simulink model "EvReferenceApplication"  (R2024b)
settings: Solver=ode23tb  StartTime=0  StopTime=2474  RelTol=1e-3  EnableMultiTasking=on
undefined symbols (not defined in the file or in its folder): SRE
undefined symbols (not defined in the file): FTP75
libraries: autolibshared x2, simulink x1, autolibutils x1
settings Model: DataDictionary=BMS_Software_DD.sldd  ModifiedByFormat=The MathWorks, Inc.  PauseTimes=0  Creator=The MathWorks, Inc.  LastModifiedBy=The MathWorks, Inc.
settings SolverCC: ZeroCrossAlgorithm=Adaptive  AlgebraicLoopSolver=TrustRegion  AutoInsertRateTranBlk=on  DecoupledContinuousIntegration=on  MinimalZcImpactIntegration=on  MaxZcPerStep=1
settings DataIOCC: SaveOutput=off  DSMLogging=off  SaveTime=off  ReturnWorkspaceOutputs=off  ReturnWorkspaceOutputsName=tp18ed42d9_4bab_49d7_8847_516cfb0e46d8
settings DebuggingCC: UnderspecifiedInitializationDetection=Classic  MergeDetectMultiDrivingBlocksExec=none  IgnoredZcDiagnostic=none  ParameterPrecisionLossMsg=none  UnconnectedInputMsg=warning  UnconnectedOutputMsg=warning  UnconnectedLineMsg=warning  PregeneratedLibrarySubsystemCodeDiagnostic=none  SubsystemReferenceDiagnosticForUnitTest=warning  ArithmeticOperatorsInVariantConditions=warning
settings ModelReferenceCC: UpdateModelReferenceTargets=IfOutOfDate  EnableRefExpFcnMdlSchedulingChecks=on  ModelReferenceMinAlgLoopOccurrences=on  PropagateSignalLabelsOutOfModel=off
settings SFSimCC: SimUseLocalCustomCode=off
settings RTWCC: RTWUseLocalCustomCode=off  GPUComputeCapability=3.5  DLArmComputeVersion=19.05
settings CodeAppCC: StateflowObjectComments=on
settings GRTTargetCC: TargetLangStandard=C89/C90 (ANSI)
settings ConfigComp: CovMetricSettings=dsw  CovSaveCumulativeToWorkspaceVar=on  CovSaveSingleToWorkspaceVar=on  CovExternalEMLEnable=off
settings SimscapeCC: SimscapeLogSimulationStatistics=on  SimscapeLogToSDI=on  SimscapeLogOpenViewer=on  SimscapeLogLimitData=off

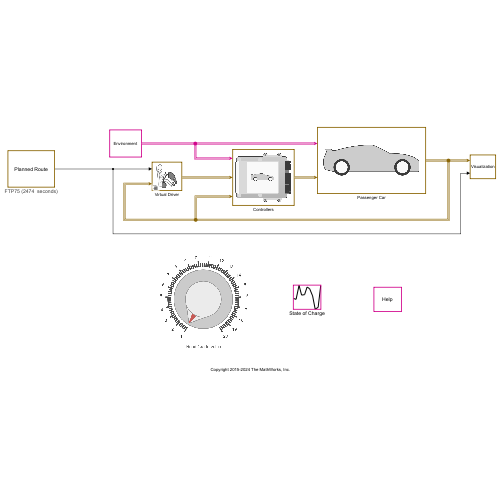
[thumbnail: Simulink's stored preview of the top-level diagram]
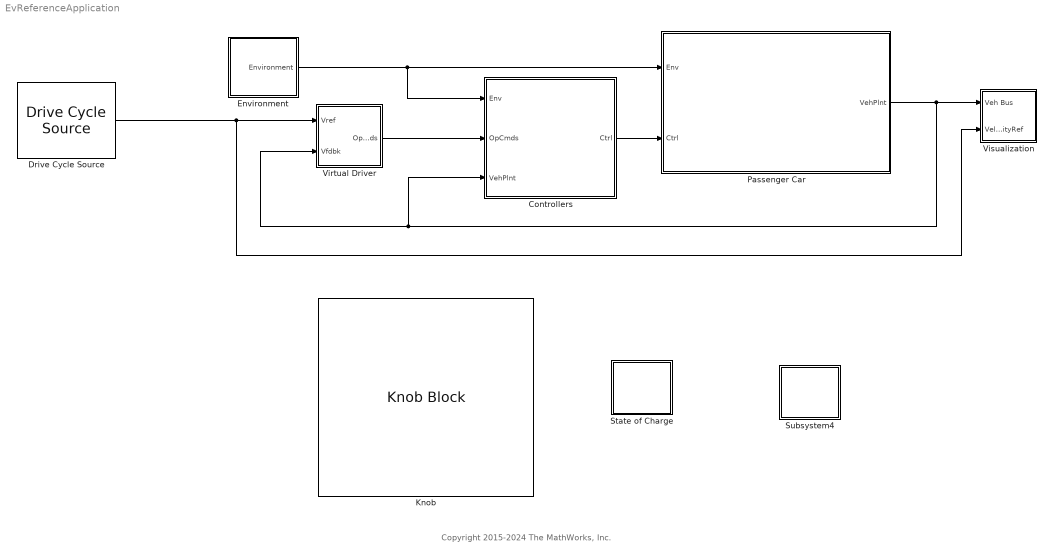
== system EvReferenceApplication ==
  note: Copyright 2015-2024 The MathWorks, Inc.
  Controllers : Subsystem
      mask Display: image('SystemControllers.png','center')
  Drive Cycle Source : autolibshared/Drive Cycle Source  cycleVar=FTP75  fileVar=L:\Bauto\matlab\test\toolbox\shared\autoblks\scenario\adac.txt  tfinal="2474  seconds"  cycleRepeat=off  outAccPort=off  outGearPort=off  gearList=No gear data  t_wot1=1  xdot_woto=0  xdot_wot1=26.8*1.1  t_wot2=30  xdot_wot2=0  t_wotend=40  srcUnit=m/s  outUnit=m/s  srcAccUnit=m/s/s  outAccUnit=m/s^2  dt=0  aMode=1  faultOption=off  velBnd=2  velBndUnit=mph  inUnit=m/s  timeBnd=1  failOption=off  stopSim=off  maxFaultCnt=10  maxFaultTime=2  maxTotFaultTime=15  traceOption=off  dtTrace=1  traceWindow=10  lastDCname=UDDS  lastOutUnit=mph  lastDT=0  lastTB=1  lastSB=2  forceCalcBound=off  mask(Drive Cycle Source){cycleVar=FTP75}
      mask prompts: cycleVar "autoblks_shared:autoblkDriveCycleSource:blkPrm_cycleVar"
      mask TypeOptions cycleVar: cycleVar
      mask DialogControl cycleVar Prompt: Drive cycle source:
      mask Display: fprintf('Planned Route');
  Environment : Subsystem
      mask Display: disp(getString(message('autoblks:autoblkVehMask:environ')))
  Knob : KnobBlock  LabelPosition=Bottom  ScaleMin=1  ScaleMax=20
  Passenger Car : Subsystem
      mask Display: image('PassengerVehicle.png','center')
  State of Charge : Subsystem
      settings: OpenFcn=open_system('EvReferenceApplication/Visualization/Scope');
      mask Display: plot(0:5:50, [.5000    0.4799    0.9047    0.6099    0.6177    0.8594    0.8055    0.5767    0.1829    0.2399    0.8865]);
  Subsystem4 : Subsystem
      settings: OpenFcn=helpview([docroot,'/toolbox/autoblks/helptargets.map'], 'ev_refapp')
      mask Display: disp(getString(message('autoblks:autoblkVehMask:help')))
  Virtual Driver : Subsystem  Variant=on  VariantControlMode=label  VariantControl=Variant1  LabelModeActiveChoice=0
      mask Display:
      | if strcmp('1',get_param(gcb,'ActiveVariant'))
      |     disp('Open Loop')
      | else
      |     image('LongitudinalDriver.png','center');
      | end
  Visualization : Subsystem
      mask Display: disp(getString(message('autoblks:autoblkVehMask:visual')))
  wires:
  Virtual Driver/1(" OpCmds") -> Controllers/2(OpCmds)
  Drive Cycle Source/1 -> Virtual Driver/1("Vref "), Visualization/2(VelocityRef)
  Environment/1(Environment) -> Controllers/1(Env), Passenger Car/1(Env)
  Controllers/1(Ctrl) -> Passenger Car/2(Ctrl)
  Passenger Car/1(VehPlnt) -> Visualization/1(Veh Bus), Virtual Driver/2("Vfdbk "), Controllers/3(VehPlnt)

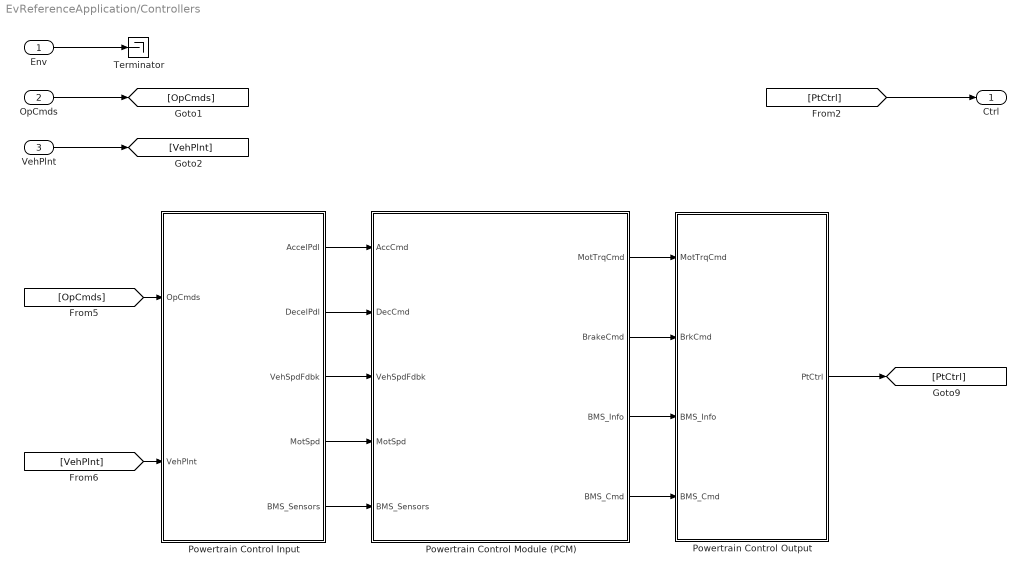
== system EvReferenceApplication/Controllers ==
  Env : Inport
  OpCmds : Inport  Port=2
  VehPlnt : Inport  Port=3
  Powertrain Control Input : Subsystem
  Powertrain Control Module (PCM) : Subsystem
  Powertrain Control Output : Subsystem
  Terminator : Terminator
  Ctrl : Outport  VectorParamsAs1DForOutWhenUnconnected=off
  wires:
  [PtCtrl] -> Ctrl/1
  Env/1 -> Terminator/1
  [OpCmds] -> Powertrain Control Input/1(OpCmds)
  Powertrain Control Output/1(PtCtrl) -> [PtCtrl]
  [VehPlnt] -> Powertrain Control Input/2(VehPlnt)
  VehPlnt/1 -> [VehPlnt]
  OpCmds/1 -> [OpCmds]
  Powertrain Control Input/1(AccelPdl) -> Powertrain Control Module (PCM)/1(AccCmd)
  Powertrain Control Input/2(DecelPdl) -> Powertrain Control Module (PCM)/2(DecCmd)
  Powertrain Control Input/3(VehSpdFdbk) -> Powertrain Control Module (PCM)/3(VehSpdFdbk)
  Powertrain Control Input/4(MotSpd) -> Powertrain Control Module (PCM)/4(MotSpd)
  Powertrain Control Module (PCM)/1(MotTrqCmd) -> Powertrain Control Output/1(MotTrqCmd)
  Powertrain Control Module (PCM)/2(BrakeCmd) -> Powertrain Control Output/2(BrkCmd)
  Powertrain Control Input/5(BMS_Sensors) -> Powertrain Control Module (PCM)/5(BMS_Sensors)
  Powertrain Control Module (PCM)/3(BMS_Info) -> Powertrain Control Output/3(BMS_Info)
  Powertrain Control Module (PCM)/4(BMS_Cmd) -> Powertrain Control Output/4(BMS_Cmd)

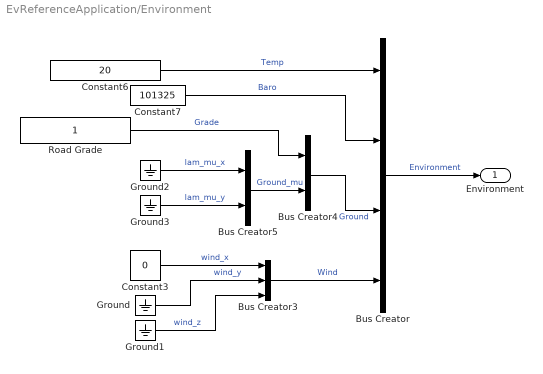
== system EvReferenceApplication/Environment ==
  Bus Creator : BusCreator  Inputs=4
  Bus Creator3 : BusCreator  Inputs=3
  Bus Creator4 : BusCreator  Inputs=2
  Bus Creator5 : BusCreator  Inputs=2
  Constant3 : Constant  Value=0
  Constant6 : Constant  Value=20
  Constant7 : Constant  Value=101325
  Ground{,1..3} (4 alike) : Ground
  Road Grade : Constant
      settings: AttributesFormatString=%<Name>
  Environment : Outport  VectorParamsAs1DForOutWhenUnconnected=off
  wires:
  Ground2/1 -> Bus Creator5/1  "lam_mu_x"
  Ground3/1 -> Bus Creator5/2  "lam_mu_y"
  Bus Creator5/1 -> Bus Creator4/2  "Ground_mu"
  Bus Creator4/1 -> Bus Creator/3  "Ground"
  Bus Creator3/1 -> Bus Creator/4  "Wind"
  Constant3/1 -> Bus Creator3/1  "wind_x"
  Ground/1 -> Bus Creator3/2  "wind_y"
  Ground1/1 -> Bus Creator3/3  "wind_z"
  Constant6/1 -> Bus Creator/1  "Temp"
  Road Grade/1 -> Bus Creator4/1  "Grade"
  Bus Creator/1 -> Environment/1  "Environment"
  Constant7/1 -> Bus Creator/2  "Baro"

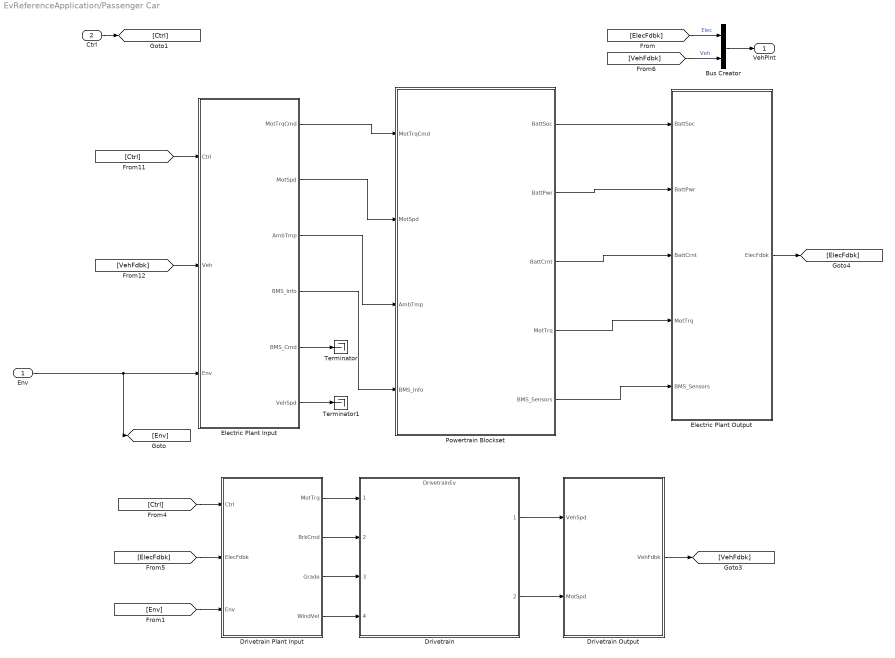
== system EvReferenceApplication/Passenger Car ==
  Env : Inport
  Ctrl : Inport  Port=2
  Bus Creator : BusCreator  Inputs=2
  Drivetrain : ModelReference  ModelNameDialog=DrivetrainEv.slx  ModelReferenceVersion=10.0
  Drivetrain Output : Subsystem
  Drivetrain Plant Input : Subsystem
  Electric Plant Input : Subsystem
  Electric Plant Output : Subsystem
  Powertrain Blockset : Subsystem  VariantControl=Powertrain Blockset
  Terminator : Terminator
  Terminator1 : Terminator
  VehPlnt : Outport  VectorParamsAs1DForOutWhenUnconnected=off
  wires:
  Ctrl/1 -> [Ctrl]
  Env/1 -> [Env], Electric Plant Input/3(Env)
  [Ctrl] -> Drivetrain Plant Input/1(Ctrl)
  Bus Creator/1 -> VehPlnt/1
  [VehFdbk] -> Bus Creator/2  "Veh"
  Drivetrain Output/1(VehFdbk) -> [VehFdbk]
  Electric Plant Output/1(ElecFdbk) -> [ElecFdbk]
  [ElecFdbk] -> Bus Creator/1  "Elec"
  [Ctrl] -> Electric Plant Input/1(Ctrl)
  [ElecFdbk] -> Drivetrain Plant Input/2(ElecFdbk)
  [VehFdbk] -> Electric Plant Input/2(Veh)
  Drivetrain Plant Input/2(BrkCmd) -> Drivetrain/2
  Drivetrain Plant Input/1(MotTrq) -> Drivetrain/1
  Drivetrain/2 -> Drivetrain Output/2(MotSpd)
  Drivetrain/1 -> Drivetrain Output/1(VehSpd)
  [Env] -> Drivetrain Plant Input/3(Env)
  Drivetrain Plant Input/3(Grade) -> Drivetrain/3
  Drivetrain Plant Input/4(WindVel) -> Drivetrain/4
  Electric Plant Input/1(MotTrqCmd) -> Powertrain Blockset/1(MotTrqCmd)
  Powertrain Blockset/2(BattPwr) -> Electric Plant Output/2(BattPwr)
  Electric Plant Input/2(MotSpd) -> Powertrain Blockset/2(MotSpd)
  Electric Plant Input/3(AmbTmp) -> Powertrain Blockset/3(AmbTmp)
  Electric Plant Input/4(BMS_Info) -> Powertrain Blockset/4(BMS_Info)
  Powertrain Blockset/1(BattSoc) -> Electric Plant Output/1(BattSoc)
  Powertrain Blockset/3(BattCrnt) -> Electric Plant Output/3(BattCrnt)
  Powertrain Blockset/4(MotTrq) -> Electric Plant Output/4(MotTrq)
  Powertrain Blockset/5(BMS_Sensors) -> Electric Plant Output/5(BMS_Sensors)
  Electric Plant Input/5(BMS_Cmd) -> Terminator/1
  Electric Plant Input/6(VehSpd) -> Terminator1/1

== system EvReferenceApplication/State of Charge ==

== system EvReferenceApplication/Subsystem4 ==

== system EvReferenceApplication/Virtual Driver ==
  note: To switch variants, right-click on this subsystem (from one level above) and chose:
      | Variant, Active choice, <your selection>
  "Vref " : Inport
  "Vfdbk " : Inport  Port=2
  Longitudinal Driver : Subsystem  VariantControl=0
      mask Display: image('LongitudinalDriver.png', 'center')
  Open Loop : Subsystem  VariantControl=1
      mask Display: disp('Open Loop')
  " OpCmds" : Outport  VectorParamsAs1DForOutWhenUnconnected=off

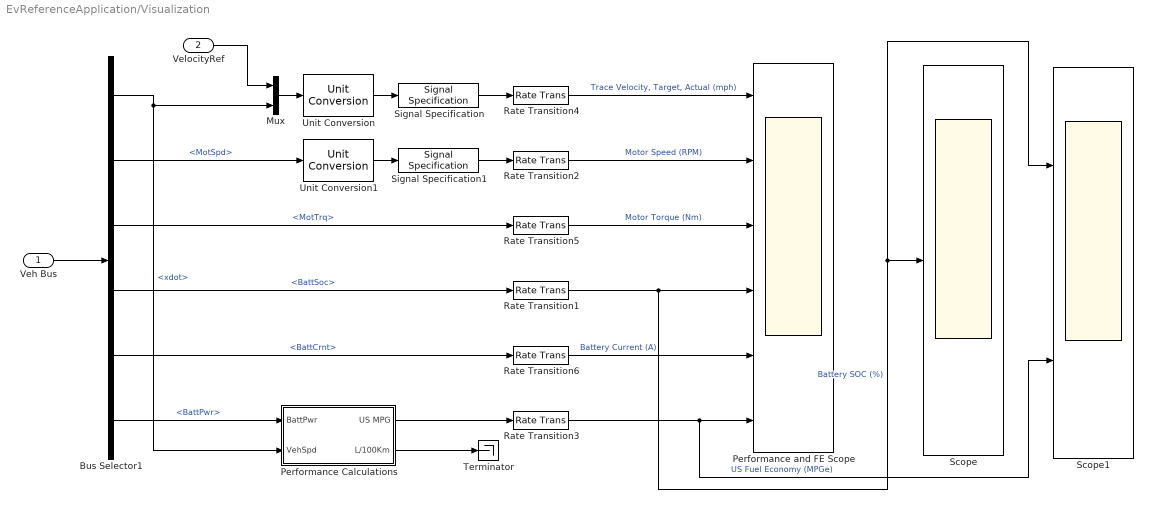
== system EvReferenceApplication/Visualization ==
  Veh Bus : Inport
  VelocityRef : Inport  Port=2
  Bus Selector1 : BusSelector  OutputSignals=Veh.xdot,Veh.MotSpd,Elec.MotTrq,Elec.BattSoc,Elec.BattCrnt,Elec.BattPwr
  Mux : Mux  Inputs=2
  Performance Calculations : Subsystem
  Performance and FE Scope : Scope  NumInputPorts=6
  Rate Transition{1..6} (6 alike) : RateTransition  Deterministic=off
  Scope : Scope
  Scope1 : Scope  NumInputPorts=2
  Signal Specification : SignalSpecification  Unit=mph
  Signal Specification1 : SignalSpecification  Unit=rpm
  Terminator : Terminator
  Unit Conversion : UnitConversion
  Unit Conversion1 : UnitConversion
  wires:
  Veh Bus/1 -> Bus Selector1/1
  Bus Selector1/1 -> Performance Calculations/2(VehSpd), Mux/2  "<xdot>"
  Mux/1 -> Unit Conversion/1
  Performance Calculations/1(US MPG) -> Rate Transition3/1
  Performance Calculations/2(L/100Km) -> Terminator/1
  Bus Selector1/4 -> Rate Transition1/1  "<BattSoc>"
  VelocityRef/1 -> Mux/1
  Rate Transition1/1 -> Scope1/1, Scope/1, Performance and FE Scope/4  "Battery SOC (%)"
  Rate Transition2/1 -> Performance and FE Scope/2  "Motor Speed (RPM)"
  Rate Transition4/1 -> Performance and FE Scope/1  "Trace Velocity, Target, Actual (mph)"
  Bus Selector1/2 -> Unit Conversion1/1  "<MotSpd>"
  Bus Selector1/6 -> Performance Calculations/1(BattPwr)  "<BattPwr>"
  Signal Specification1/1 -> Rate Transition2/1
  Bus Selector1/3 -> Rate Transition5/1  "<MotTrq>"
  Rate Transition5/1 -> Performance and FE Scope/3  "Motor Torque (Nm)"
  Rate Transition6/1 -> Performance and FE Scope/5  "Battery Current (A)"
  Bus Selector1/5 -> Rate Transition6/1  "<BattCrnt>"
  Rate Transition3/1 -> Scope1/2, Performance and FE Scope/6  "US Fuel Economy (MPGe)"
  Unit Conversion/1 -> Signal Specification/1
  Signal Specification/1 -> Rate Transition4/1
  Unit Conversion1/1 -> Signal Specification1/1

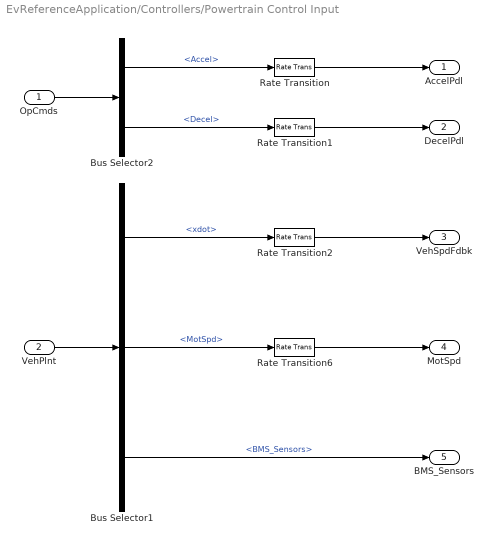
== system EvReferenceApplication/Controllers/Powertrain Control Input ==
  OpCmds : Inport
  VehPlnt : Inport  Port=2
  Bus Selector1 : BusSelector  OutputSignals=Veh.xdot,Veh.MotSpd,Elec.BMS_Sensors
  Bus Selector2 : BusSelector  OutputSignals=Accel,Decel
  Rate Transition{,1..2,6} (4 alike) : RateTransition  Deterministic=off
  AccelPdl : Outport  VectorParamsAs1DForOutWhenUnconnected=off
  DecelPdl : Outport  Port=2  VectorParamsAs1DForOutWhenUnconnected=off
  VehSpdFdbk : Outport  Port=3  VectorParamsAs1DForOutWhenUnconnected=off
  MotSpd : Outport  Port=4  VectorParamsAs1DForOutWhenUnconnected=off
  BMS_Sensors : Outport  Port=5  OutDataTypeStr=Bus: Sensors  VectorParamsAs1DForOutWhenUnconnected=off
  wires:
  OpCmds/1 -> Bus Selector2/1
  VehPlnt/1 -> Bus Selector1/1
  Bus Selector2/1 -> Rate Transition/1  "<Accel>"
  Bus Selector2/2 -> Rate Transition1/1  "<Decel>"
  Bus Selector1/1 -> Rate Transition2/1  "<xdot>"
  Bus Selector1/2 -> Rate Transition6/1  "<MotSpd>"
  Rate Transition/1 -> AccelPdl/1
  Rate Transition1/1 -> DecelPdl/1
  Rate Transition2/1 -> VehSpdFdbk/1
  Rate Transition6/1 -> MotSpd/1
  Bus Selector1/3 -> BMS_Sensors/1  "<BMS_Sensors>"

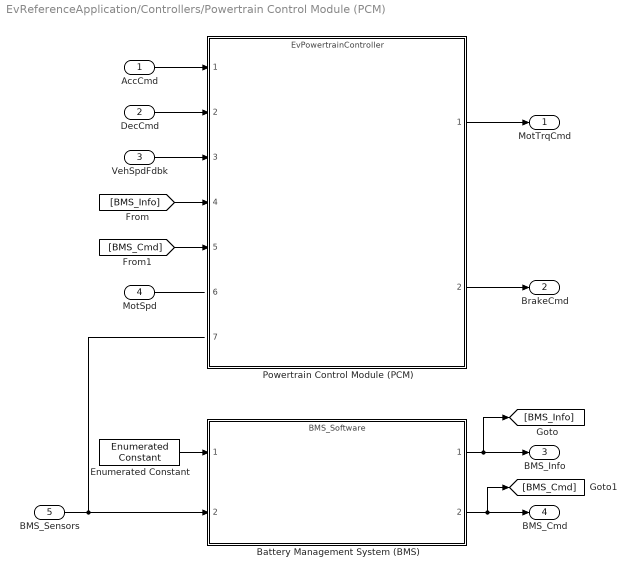
== system EvReferenceApplication/Controllers/Powertrain Control Module (PCM) ==
  AccCmd : Inport
  DecCmd : Inport  Port=2
  VehSpdFdbk : Inport  Port=3
  MotSpd : Inport  Port=4
  BMS_Sensors : Inport  Port=5  OutDataTypeStr=Bus: Sensors
  Battery Management System (BMS) : ModelReference  ModelNameDialog=BMS_Software.slx  ModelReferenceVersion=8.0
  Enumerated Constant : simulink/Sources/Enumerated Constant  OutDataTypeStr=Enum: SRE  Value=SRE.Driving  SampleTime=inf
  Powertrain Control Module (PCM) : ModelReference  ModelNameDialog=EvPowertrainController.slx  ModelReferenceVersion=8.0
  MotTrqCmd : Outport
  BrakeCmd : Outport  Port=2
  BMS_Info : Outport  Port=3  OutDataTypeStr=Bus: BMS_Info
  BMS_Cmd : Outport  Port=4  OutDataTypeStr=Bus: BMS_Cmd
  wires:
  DecCmd/1 -> Powertrain Control Module (PCM)/2
  Powertrain Control Module (PCM)/1 -> MotTrqCmd/1
  [BMS_Info] -> Powertrain Control Module (PCM)/4
  MotSpd/1 -> ?
  VehSpdFdbk/1 -> Powertrain Control Module (PCM)/3
  AccCmd/1 -> Powertrain Control Module (PCM)/1
  Powertrain Control Module (PCM)/2 -> BrakeCmd/1
  Enumerated Constant/1 -> Battery Management System (BMS)/1
  Battery Management System (BMS)/1 -> [BMS_Info], BMS_Info/1
  Battery Management System (BMS)/2 -> [BMS_Cmd], BMS_Cmd/1
  BMS_Sensors/1 -> Battery Management System (BMS)/2
  [BMS_Cmd] -> Powertrain Control Module (PCM)/5

== system EvReferenceApplication/Controllers/Powertrain Control Output ==
  MotTrqCmd : Inport
  BrkCmd : Inport  Port=2
  BMS_Info : Inport  Port=3  OutDataTypeStr=Bus: BMS_Info
  BMS_Cmd : Inport  Port=4  OutDataTypeStr=Bus: BMS_Cmd
  Bus Creator : BusCreator  Inputs=4
  PtCtrl : Outport  VectorParamsAs1DForOutWhenUnconnected=off
  wires:
  BrkCmd/1 -> Bus Creator/2  "BrkCmd"
  Bus Creator/1 -> PtCtrl/1  "PtCtrl"
  MotTrqCmd/1 -> Bus Creator/1  "MotTrqCmd"
  BMS_Info/1 -> Bus Creator/3  "BMS_Info"
  BMS_Cmd/1 -> Bus Creator/4  "BMS_Cmd"

== system EvReferenceApplication/Passenger Car/Drivetrain Output ==
  VehSpd : Inport
  MotSpd : Inport  Port=2
  Bus Creator1 : BusCreator  Inputs=2
  VehFdbk : Outport  VectorParamsAs1DForOutWhenUnconnected=off
  wires:
  Bus Creator1/1 -> VehFdbk/1  "VehFdbk"
  VehSpd/1 -> Bus Creator1/1
  MotSpd/1 -> Bus Creator1/2  "MotSpd"

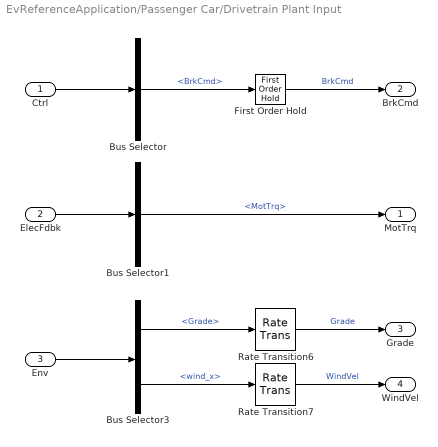
== system EvReferenceApplication/Passenger Car/Drivetrain Plant Input ==
  Ctrl : Inport
  ElecFdbk : Inport  Port=2
  Env : Inport  Port=3
  Bus Selector : BusSelector  OutputSignals=BrkCmd
  Bus Selector1 : BusSelector  OutputSignals=MotTrq
  Bus Selector3 : BusSelector  OutputSignals=Ground.Grade,Wind.wind_x
  First Order Hold : FirstOrderHold  ErrorTolerance=inf
  Rate Transition6 : RateTransition  Deterministic=off
  Rate Transition7 : RateTransition  Deterministic=off
  MotTrq : Outport  VectorParamsAs1DForOutWhenUnconnected=off
  BrkCmd : Outport  Port=2  VectorParamsAs1DForOutWhenUnconnected=off
  Grade : Outport  Port=3  VectorParamsAs1DForOutWhenUnconnected=off
  WindVel : Outport  Port=4  VectorParamsAs1DForOutWhenUnconnected=off
  wires:
  Ctrl/1 -> Bus Selector/1
  Bus Selector/1 -> First Order Hold/1  "<BrkCmd>"
  First Order Hold/1 -> BrkCmd/1  "BrkCmd"
  ElecFdbk/1 -> Bus Selector1/1
  Bus Selector1/1 -> MotTrq/1  "<MotTrq>"
  Env/1 -> Bus Selector3/1
  Rate Transition6/1 -> Grade/1  "Grade"
  Rate Transition7/1 -> WindVel/1  "WindVel"
  Bus Selector3/1 -> Rate Transition6/1  "<Grade>"
  Bus Selector3/2 -> Rate Transition7/1  "<wind_x>"

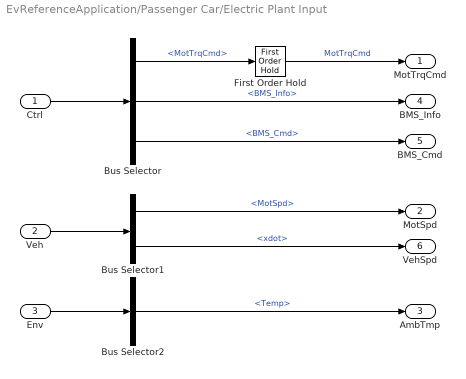
== system EvReferenceApplication/Passenger Car/Electric Plant Input ==
  Ctrl : Inport
  Veh : Inport  Port=2
  Env : Inport  Port=3
  Bus Selector : BusSelector  OutputSignals=MotTrqCmd,BMS_Info,BMS_Cmd
  Bus Selector1 : BusSelector  OutputSignals=MotSpd,xdot
  Bus Selector2 : BusSelector  OutputSignals=Temp
  First Order Hold : FirstOrderHold  ErrorTolerance=inf
  MotTrqCmd : Outport  VectorParamsAs1DForOutWhenUnconnected=off
  MotSpd : Outport  Port=2  VectorParamsAs1DForOutWhenUnconnected=off
  AmbTmp : Outport  Port=3  VectorParamsAs1DForOutWhenUnconnected=off
  BMS_Info : Outport  Port=4  OutDataTypeStr=Bus: BMS_Info  VectorParamsAs1DForOutWhenUnconnected=off
  BMS_Cmd : Outport  Port=5  OutDataTypeStr=Bus: BMS_Cmd  VectorParamsAs1DForOutWhenUnconnected=off
  VehSpd : Outport  Port=6  VectorParamsAs1DForOutWhenUnconnected=off
  wires:
  First Order Hold/1 -> MotTrqCmd/1  "MotTrqCmd"
  Ctrl/1 -> Bus Selector/1
  Bus Selector/1 -> First Order Hold/1  "<MotTrqCmd>"
  Veh/1 -> Bus Selector1/1
  Bus Selector1/1 -> MotSpd/1  "<MotSpd>"
  Env/1 -> Bus Selector2/1
  Bus Selector2/1 -> AmbTmp/1  "<Temp>"
  Bus Selector/2 -> BMS_Info/1  "<BMS_Info>"
  Bus Selector/3 -> BMS_Cmd/1  "<BMS_Cmd>"
  Bus Selector1/2 -> VehSpd/1  "<xdot>"

== system EvReferenceApplication/Passenger Car/Electric Plant Output ==
  BattSoc : Inport
  BattPwr : Inport  Port=2
  BattCrnt : Inport  Port=3
  MotTrq : Inport  Port=4
  BMS_Sensors : Inport  Port=5  OutDataTypeStr=Bus: Sensors
  Bus Creator1 : BusCreator  Inputs=5
  ElecFdbk : Outport  VectorParamsAs1DForOutWhenUnconnected=off
  wires:
  Bus Creator1/1 -> ElecFdbk/1  "ElecFdbk"
  BattPwr/1 -> Bus Creator1/2
  BattCrnt/1 -> Bus Creator1/3
  MotTrq/1 -> Bus Creator1/4
  BMS_Sensors/1 -> Bus Creator1/5
  BattSoc/1 -> Bus Creator1/1

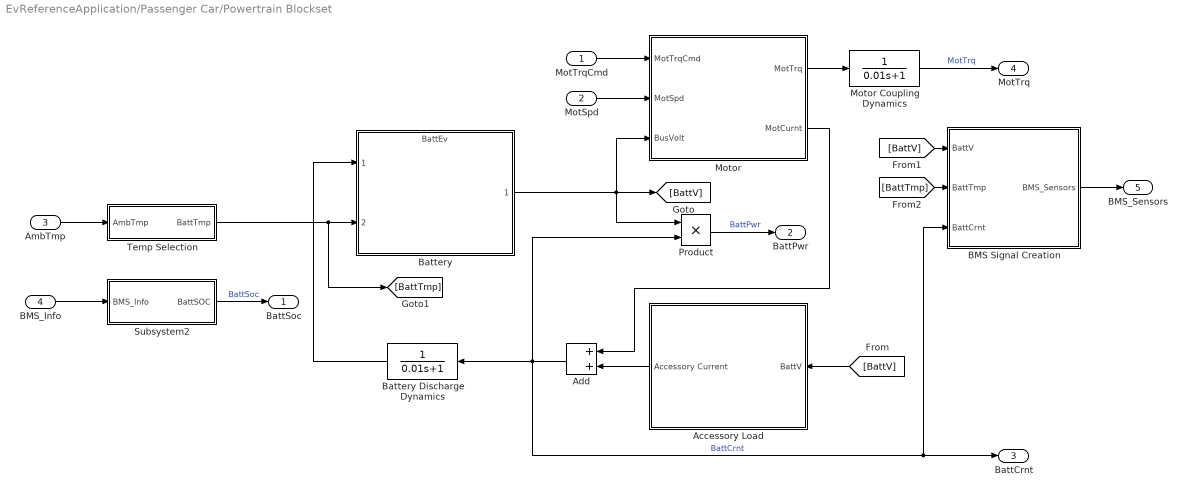
== system EvReferenceApplication/Passenger Car/Powertrain Blockset ==
  MotTrqCmd : Inport
  MotSpd : Inport  Port=2
  AmbTmp : Inport  Port=3
  BMS_Info : Inport  Port=4  OutDataTypeStr=Bus: BMS_Info
  Accessory Load : Subsystem
  Add : Sum
  BMS Signal Creation : Subsystem
  Battery : ModelReference  ModelNameDialog=BattEv.slx  SimulationMode=Normal  ModelReferenceVersion=12.4
  Battery Discharge Dynamics : TransferFcn  Denominator=[0.01 1]
  Motor : Subsystem  Variant=on  VariantControlMode=label  LabelModeActiveChoice=MotGenEvMapped
  Motor Coupling Dynamics : TransferFcn  Denominator=[0.01 1]
  Product : Product
  Subsystem2 : Subsystem
  Temp Selection : Subsystem
  BattSoc : Outport
  BattPwr : Outport  Port=2  VectorParamsAs1DForOutWhenUnconnected=off
  BattCrnt : Outport  Port=3  VectorParamsAs1DForOutWhenUnconnected=off
  MotTrq : Outport  Port=4  VectorParamsAs1DForOutWhenUnconnected=off
  BMS_Sensors : Outport  Port=5  OutDataTypeStr=Bus: Sensors  VectorParamsAs1DForOutWhenUnconnected=off
  wires:
  MotTrqCmd/1 -> Motor/1(MotTrqCmd)
  MotSpd/1 -> Motor/2(MotSpd)
  Battery/1 -> Product/1, Motor/3(BusVolt), [BattV]
  Product/1 -> BattPwr/1  "BattPwr"
  Battery Discharge Dynamics/1 -> Battery/1
  Motor/1(MotTrq) -> Motor Coupling Dynamics/1
  Motor Coupling Dynamics/1 -> MotTrq/1  "MotTrq"
  Accessory Load/1(Accessory Current) -> Add/2
  Motor/2(MotCurnt) -> Add/1
  [BattV] -> Accessory Load/1(BattV)
  Add/1 -> Battery Discharge Dynamics/1, BattCrnt/1, BMS Signal Creation/3(BattCrnt), Product/2  "BattCrnt"
  [BattV] -> BMS Signal Creation/1(BattV)
  [BattTmp] -> BMS Signal Creation/2(BattTmp)
  BMS Signal Creation/1(BMS_Sensors) -> BMS_Sensors/1
  AmbTmp/1 -> Temp Selection/1(AmbTmp)
  Temp Selection/1(BattTmp) -> [BattTmp], Battery/2
  BMS_Info/1 -> Subsystem2/1(BMS_Info)
  Subsystem2/1(BattSOC) -> BattSoc/1  "BattSoc"

== system EvReferenceApplication/Virtual Driver/Longitudinal Driver ==
  Vref : Inport
  Vfdbk : Inport  Port=2
  Bus Selector : BusSelector  OutputSignals=Veh.xdot
  Ground : Ground
  Longitudinal Driver Model : autolibshared/Longitudinal Driver  extAccelOvr=off  extDecelOvr=off  extAccelHld=off  extDecelHld=off  extAccelZero=off  extDecelZero=off  cntrlType=Predictive  shftType=Reverse, Neutral, Drive  velUnits=m/s  gearOut=off  Kp=1  Ki=1  Kff=0  Kg=0  VehVelVec=[0 100]  KffVec=[.1 .1]  KpVec=[10 10]  KiVec=[5 5]  KgVec=[0 0]  m=1645  Kpt=450*9.04/0.324  tau=0.12  L=4  aR=30.3/3875  bR=0.21290*4.44822/0.44704  cR=0.01278*4.44822/0.44704^2  g=9.81  vnom=1  Kaw=0  tauerr=0  tauPt=2  GearInit=0  tShift=.1  pdlVec=[0.1 0.4 0.5 0.9]  upShftTbl=[-1 12.9375 26.4375 39.9375 51.18749999999999 62.4375 72.84375 83.25;-1 16.3125 29.8125 43.3125 54.5624 65.8125 76.78125 87.75;-1 19.6875 33.1875 46.68749999999999 57.9375 69.1875 80.71875 92.25;-1 33 52.5 77.25 100.5 138.75 161.875 185]  dwnShftTbl=[1 9.5625 23.0625 36.5625 47.8125 59.0625 68.90625 78.75;1 12.9375 26.4375 39.9375 51.18749999999999 62.4375 72.84375 83.25;1 16.3125 29.8125 43.3125 54.562499 65.8125 76.78125 87.75;1 19.6875 33.1875 46.68749999999999 57.9375 69.1875 80.71875 92.25]  tClutch=.5  tRev=.5  tPark=120  aMode=1  UpGearVec="[0  1  2  3  4  5  6  7]"  DownGearVec="[1  2  3  4  5  6  7  8]"
  Terminator : Terminator
  Terminator1 : Terminator
  OpCmds : Outport  VectorParamsAs1DForOutWhenUnconnected=off
  wires:
  Bus Selector/1 -> Longitudinal Driver Model/2  "<xdot>"
  Vref/1 -> Longitudinal Driver Model/1  "xdotref"
  Vfdbk/1 -> Bus Selector/1
  Longitudinal Driver Model/2 -> Terminator/1  "Acc"
  Longitudinal Driver Model/3 -> Terminator1/1  "Dec"
  Ground/1 -> Longitudinal Driver Model/3
  Longitudinal Driver Model/1 -> OpCmds/1  "Info"

== system EvReferenceApplication/Virtual Driver/Open Loop ==
  note: This subsystem is provided to disable the driver subsystem and expose the driver interface.
      |
      | The interface can:
      | - be connected with dashboard UI blocks or 3rd party hardware
      | - provide application specific pre-programmed event or time based signals
      | - be driven by recorded operator signals for tuning, troubleshooting and model validation
  Bus Creator2 : BusCreator  Inputs=8
  Constant{1..4} (4 alike) : Constant  Value=0
  Ground{,1..3} (4 alike) : Ground
  OpCmds : Outport  VectorParamsAs1DForOutWhenUnconnected=off
  wires:
  Ground3/1 -> Bus Creator2/8  "ErrMin"
  Ground1/1 -> Bus Creator2/6  "ErrSqrSum"
  Bus Creator2/1 -> OpCmds/1  "Info"
  Ground2/1 -> Bus Creator2/7  "ErrMax"
  Constant1/1 -> Bus Creator2/1  "Accel"
  Constant3/1 -> Bus Creator2/3  "Gear"
  Constant2/1 -> Bus Creator2/2  "Decel"
  Ground/1 -> Bus Creator2/5  "Err"
  Constant4/1 -> Bus Creator2/4  "Clutch"

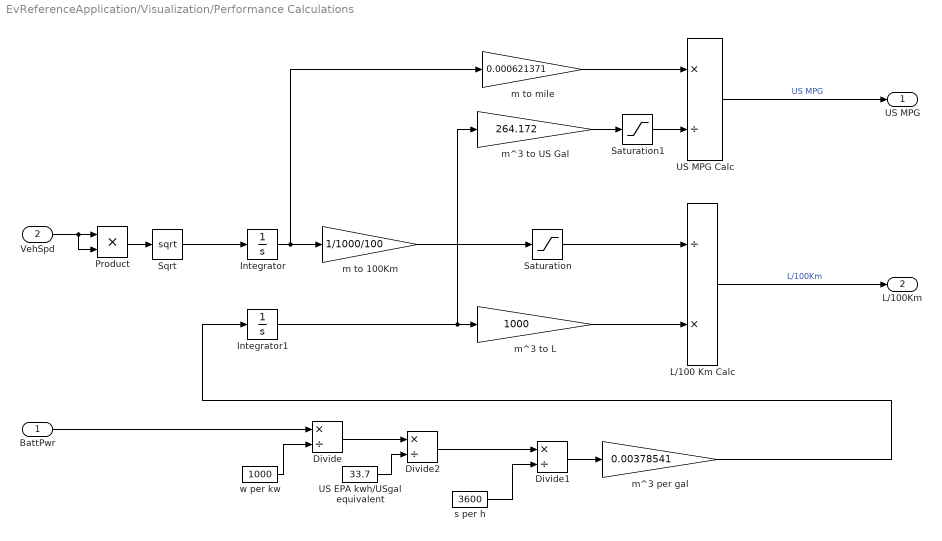
== system EvReferenceApplication/Visualization/Performance Calculations ==
  BattPwr : Inport
  VehSpd : Inport  Port=2
  Divide : Product  Inputs=*/
  Divide1 : Product  Inputs=*/
  Divide2 : Product  Inputs=*/
  Integrator : Integrator
  Integrator1 : Integrator
  L/100 Km Calc : Product  Inputs=/*
  Product : Product
  Saturation : Saturate  UpperLimit=Inf  LowerLimit=0.001  ZeroCross=off
  Saturation1 : Saturate  UpperLimit=Inf  LowerLimit=1e-3  ZeroCross=off
  Sqrt : Sqrt
  US EPA kwh/USgal equivalent : Constant  Value=33.7
  US MPG Calc : Product  Inputs=*/
  m to 100Km : Gain  Gain=1/1000/100
  m to mile : Gain  Gain=0.000621371
  m^3 per gal : Gain  Gain=0.00378541
  m^3 to L : Gain  Gain=1000
  m^3 to US Gal : Gain  Gain=264.172
  s per h : Constant  Value=3600
  w per kw : Constant  Value=1000
  US MPG : Outport  VectorParamsAs1DForOutWhenUnconnected=off
  L/100Km : Outport  Port=2  VectorParamsAs1DForOutWhenUnconnected=off
  wires:
  m^3 to US Gal/1 -> Saturation1/1
  m^3 to L/1 -> L/100 Km Calc/2
  Integrator/1 -> m to mile/1, m to 100Km/1
  m to mile/1 -> US MPG Calc/1
  Integrator1/1 -> m^3 to US Gal/1, m^3 to L/1
  Saturation/1 -> L/100 Km Calc/1
  m to 100Km/1 -> Saturation/1
  L/100 Km Calc/1 -> L/100Km/1  "L/100Km"
  Saturation1/1 -> US MPG Calc/2
  US MPG Calc/1 -> US MPG/1  "US MPG"
  w per kw/1 -> Divide/2
  Divide/1 -> Divide2/1
  Divide2/1 -> Divide1/1
  s per h/1 -> Divide1/2
  Divide1/1 -> m^3 per gal/1
  m^3 per gal/1 -> Integrator1/1
  US EPA kwh/USgal equivalent/1 -> Divide2/2
  BattPwr/1 -> Divide/1
  Sqrt/1 -> Integrator/1
  Product/1 -> Sqrt/1
  VehSpd/1 -> Product/2, Product/1

== system EvReferenceApplication/Passenger Car/Powertrain Blockset/Accessory Load ==
  BattV : Inport
  Accessory Load W : Constant  Value=0
  Divide : Product  Inputs=*/
  div0protect - poly : autolibutils/div0protect - poly  thresh=.01  ZeroCross=off  ZeroCross1=off  aMode=aMode
  Accessory Current : Outport
  wires:
  BattV/1 -> div0protect - poly/1
  Accessory Load W/1 -> Divide/1
  Divide/1 -> Accessory Current/1
  div0protect - poly/1 -> Divide/2

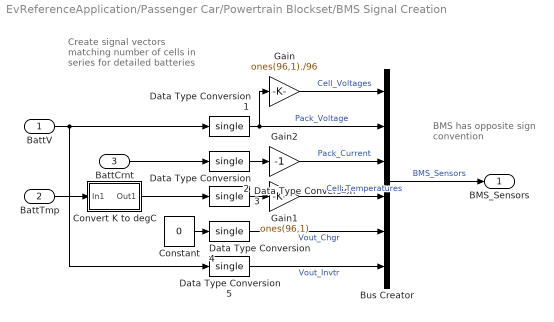
== system EvReferenceApplication/Passenger Car/Powertrain Blockset/BMS Signal Creation ==
  note: Create signal vectors
      | matching number of
      | cells in series for
      | detailed batteries
  note: BMS has opposite
      | sign convention
  BattV : Inport
  BattTmp : Inport  Port=2
  BattCrnt : Inport  Port=3
  Bus Creator : BusCreator  Inputs=6  OutDataTypeStr=Bus: Sensors  NonVirtualBus=on
      settings: InheritFromInputs=off
  Constant : Constant  Value=0
  Convert K to degC : Subsystem
  Data Type Conversion{1..5} (5 alike) : DataTypeConversion  OutDataTypeStr=single  SaturateOnIntegerOverflow=off  RndMeth=Floor
  Gain : Gain  Gain=ones(96,1)./96
  Gain1 : Gain  Gain=ones(96,1)
  Gain2 : Gain  Gain=-1
  BMS_Sensors : Outport
  wires:
  Gain1/1 -> Bus Creator/4  "Cell_Temperatures"
  Data Type Conversion4/1 -> Bus Creator/5  "Vout_Chgr"
  Gain2/1 -> Bus Creator/3  "Pack_Current"
  Data Type Conversion5/1 -> Bus Creator/6  "Vout_Invtr"
  Data Type Conversion2/1 -> Gain2/1
  Gain/1 -> Bus Creator/1  "Cell_Voltages"
  Data Type Conversion3/1 -> Gain1/1
  Data Type Conversion1/1 -> Gain/1, Bus Creator/2  "Pack_Voltage"
  BattTmp/1 -> Convert K to degC/1(In1)
  BattCrnt/1 -> Data Type Conversion2/1
  Constant/1 -> Data Type Conversion4/1
  BattV/1 -> Data Type Conversion1/1, Data Type Conversion5/1
  Bus Creator/1 -> BMS_Sensors/1  "BMS_Sensors"
  Convert K to degC/1(Out1) -> Data Type Conversion3/1

== system EvReferenceApplication/Passenger Car/Powertrain Blockset/Motor ==
  MotTrqCmd : Inport
  MotSpd : Inport  Port=2
  BusVolt : Inport  Port=3
  MotGenEvDynamic : ModelReference  ModelNameDialog=MotGenEvDynamic.slx  SimulationMode=Normal  VariantControl=MotGenEvDynamic  ModelReferenceVersion=11.0
  MotGenEvMapped : ModelReference  ModelNameDialog=MotGenEvMapped.slx  SimulationMode=Normal  VariantControl=MotGenEvMapped  ModelReferenceVersion=9.0
  MotTrq : Outport  VectorParamsAs1DForOutWhenUnconnected=off
  MotCurnt : Outport  Port=2  VectorParamsAs1DForOutWhenUnconnected=off

== system EvReferenceApplication/Passenger Car/Powertrain Blockset/Subsystem2 ==
  In Bus Element : Inport  PortName=BMS_Info  Element=SOC
  Bus Selector : BusSelector  OutputSignals=SOC_CC
  Data Type Conversion : DataTypeConversion  SaturateOnIntegerOverflow=off  RndMeth=Floor
  Rate Transition : RateTransition  Commented=through
  convert2percent : Gain  Gain=100
  BattSOC : Outport
  wires:
  In Bus Element/1 -> Bus Selector/1
  convert2percent/1 -> Data Type Conversion/1
  Bus Selector/1 -> convert2percent/1  "<SOC_CC>"
  Data Type Conversion/1 -> Rate Transition/1
  Rate Transition/1 -> BattSOC/1

== system EvReferenceApplication/Passenger Car/Powertrain Blockset/Temp Selection ==
  AmbTmp : Inport
  Constant : Constant  Value=25
  Convert degC to K : Subsystem
  Convert degC to K1 : Subsystem
  Manual Switch : ManualSwitch
  BattTmp : Outport
  wires:
  Manual Switch/1 -> BattTmp/1
  Constant/1 -> Convert degC to K/1(In1)
  Convert degC to K/1(Out1) -> Manual Switch/2
  AmbTmp/1 -> Convert degC to K1/1(In1)
  Convert degC to K1/1(Out1) -> Manual Switch/1

== system EvReferenceApplication/Passenger Car/Powertrain Blockset/BMS Signal Creation/Convert K to degC ==
  In1 : Inport
  Constant1 : Constant  Value=273.15
  Sum : Sum  Inputs=+-
  Out1 : Outport
  wires:
  In1/1 -> Sum/1
  Constant1/1 -> Sum/2
  Sum/1 -> Out1/1

== system EvReferenceApplication/Passenger Car/Powertrain Blockset/Temp Selection/Convert degC to K ==
  In1 : Inport
  Constant1 : Constant  Value=273.15
  Sum : Sum
  Out1 : Outport
  wires:
  In1/1 -> Sum/1
  Constant1/1 -> Sum/2
  Sum/1 -> Out1/1

== system EvReferenceApplication/Passenger Car/Powertrain Blockset/Temp Selection/Convert degC to K1 ==
  In1 : Inport
  Constant1 : Constant  Value=273.15
  Sum : Sum
  Out1 : Outport
  wires:
  In1/1 -> Sum/1
  Constant1/1 -> Sum/2
  Sum/1 -> Out1/1
